simulink model "PSK"  (Simulink 8.2)
settings: Solver=ode45  StartTime=0.0  StopTime=10  RelTol=1e-3
libraries: dsparch4 x2, commchan3 x1, commrandsrc2 x1, commsink2 x1, dspsigops x1
settings Model: Creator=Yi_Liu  LastModifiedBy=Yi_Liu
settings DataIOCC: SignalLoggingSaveFormat=Dataset
settings OptimizationCC: ExpressionDepthLimit=128
settings DebuggingCC: FcnCallInpInsideContextMsg=EnableAllAsError  StateNameClashWarn=none
settings GRTTargetCC: CombineOutputUpdateFcns=on  GRTInterface=off

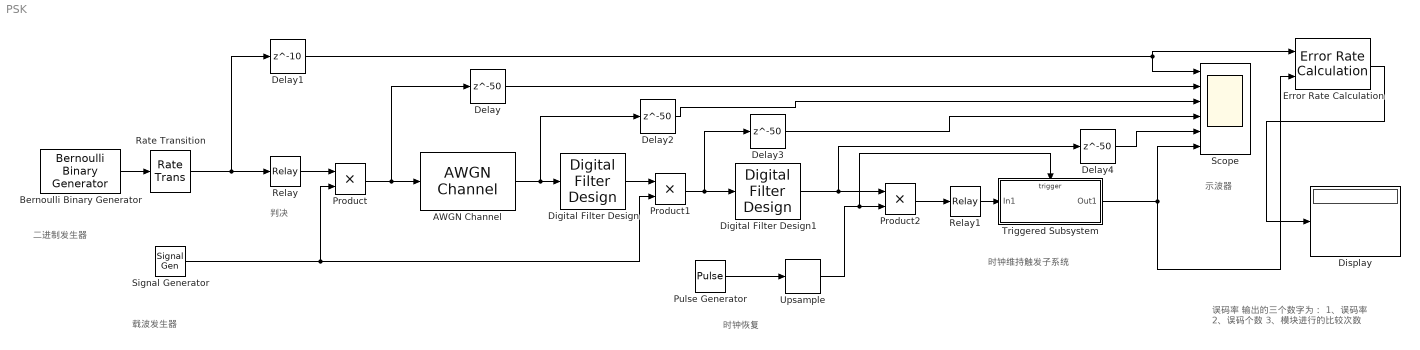
== system PSK ==
  note: 误码率
      | 输出的三个数字为：
      | 1、误码率
      | 2、误码个数
      | 3、模块进行的比较次数
  note: 示波器
  note: 时钟维持触发子系统
  note: 时钟恢复
  note: 判决
  note: 载波发生器
  note: 二进制发生器
  AWGN Channel : commchan3/AWGN Channel  InputProcessing=Columns as channels (frame based)  seed=67  noiseMode=Variance from mask  EbNodB=10  EsNodB=10  SNRdB=50  bitsPerSym=1  Ps=1  Tsym=1  variance=0.01
  Bernoulli Binary Generator : commrandsrc2/Bernoulli Binary Generator  P=0.5  seed=128  Ts=1/100  frameBased=off  sampPerFrame=1  orient=off  outDataType=double
  Delay{,2..4} (4 alike) : Delay  DelayLength=50  InitialCondition=0  SampleTime=1/50000
  Delay1 : Delay  DelayLength=10  InitialCondition=0  SampleTime=1/10000
  Digital Filter Design : dsparch4/Digital Filter Design  mwdsp_browser_bugfix_var=off
  Digital Filter Design1 : dsparch4/Digital Filter Design  mwdsp_browser_bugfix_var=off
  Display : Display
  Error Rate Calculation : commsink2/Error Rate Calculation  N=0  st_delay=0  cp_mode=Entire frame  subframe=[]  PMode=Port  WsName=ErrorVec  RsMode2=off  stop=off  numErr=100  maxBits=1e6
  Product : Product
  Product1 : Product
  Product2 : Product
  Pulse Generator : DiscretePulseGenerator  Period=10  PulseWidth=5  SampleTime=1/10000
  Rate Transition : RateTransition  OutPortSampleTime=1/1000
  Relay : Relay  OnSwitchValue=0.5  OffSwitchValue=0.5  OffOutputValue=-1  SampleTime=0.001
  Relay1 : Relay  OnSwitchValue=0  OffSwitchValue=0  SampleTime=0.001
  Scope : Scope  NumInputPorts=6
      settings: TimeRange=10  YMin=-2~-5~-5~-5~-5~-2  YMax=2~5~5~5~5~2
  Signal Generator : SignalGenerator  Frequency=2*pi*1000  Units=rad/sec
  Triggered Subsystem : Subsystem  TreatAsAtomicUnit=on
  Upsample : dspsigops/Upsample  N=10  phase=0  RateOptions=Allow multirate processing  ic=0  mode=Unused parameter value
  wires:
  Bernoulli Binary Generator/1 -> Rate Transition/1
  Rate Transition/1 -> Delay1/1, Relay/1
  Relay/1 -> Product/1
  Product/1 -> Delay/1, AWGN Channel/1
  AWGN Channel/1 -> Digital Filter Design/1, Delay2/1
  Digital Filter Design/1 -> Product1/1
  Signal Generator/1 -> Product1/2, Product/2
  Product1/1 -> Digital Filter Design1/1, Delay3/1
  Relay1/1 -> Triggered Subsystem/1(In1)
  Product2/1 -> Relay1/1
  Digital Filter Design1/1 -> Delay4/1, Product2/1
  Pulse Generator/1 -> Upsample/1
  Upsample/1 -> Triggered Subsystem/Trigger, Product2/2
  Triggered Subsystem/1(Out1) -> Error Rate Calculation/2, Scope/6
  Error Rate Calculation/1 -> Display/1
  Delay/1 -> Scope/2
  Delay1/1 -> Scope/1, Error Rate Calculation/1
  Delay2/1 -> Scope/3
  Delay3/1 -> Scope/4
  Delay4/1 -> Scope/5

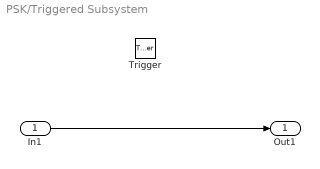
== system PSK/Triggered Subsystem ==
  In1 : Inport
  Trigger : TriggerPort
  Out1 : Outport
  wires:
  In1/1 -> Out1/1
